simulink subsystem "Thermofluids_GS"  (R2025a)
settings: Solver=VariableStepAuto  StartTime=0.0  StopTime=10.0  RelTol=1e-3
settings Model: Creator=Adam  LastModifiedBy=MW

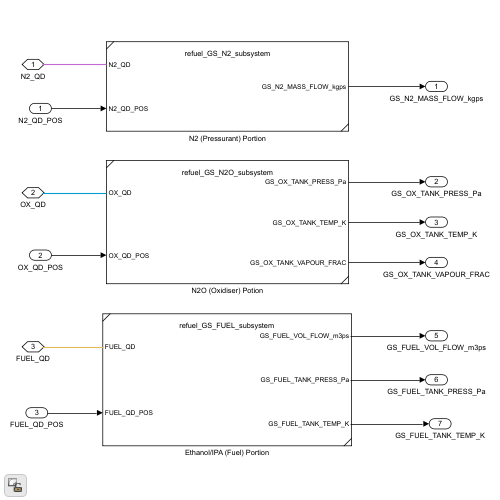
[thumbnail: Simulink's stored preview of the top-level diagram]
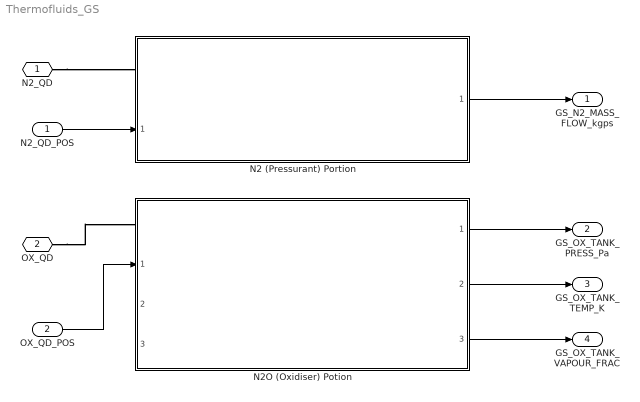
== system Thermofluids_GS ==
  N2_QD_POS : Inport
  OX_QD_POS : Inport  Port=2
  N2 (Pressurant) Portion : Subsystem  ReferencedSubsystem=refuel_GS_N2_subsystem
      settings: PortSchema="{\"entries\":[{\"content\":{\"sides\":[{\"content\":{\"connectorIds\":[\"LConn1\",\"In1\"]},\"type\":\"ConnectorPlacement.EquallySpacedRectSide\",\"uuid\":\"80a1b4a4-a86f-460b-b4b9-f1e834cc0a6f\"},{\"content\":{\"connectorIds\":[\"Out1\"],\"side\":\"RIGHT\"},\"type\":\"ConnectorPlacement.EquallySpacedRectSide\",\"uuid\":\"7a691a14-4b0a-4077-9abf-8e4fa479ec3d\"},{\"content\":{\"side\":\"TOP\"},\"type\":\"ConnectorPlacement.EquallySpacedRectSide\",\"uuid\":\"b8dd7e20-acb6-44c1-83ed-0b89a390ff72\"}]},\"type\":\"ConnectorPlacement.EquallySpacedConnector\",\"uuid\":\"2e88b817-b41b-4786-aed1-deff05c2a84d\"}],\"packageUris\":[\"http://schema.mathworks.com/mf0/Connector/R2020b\"],\"version\":\"1.0\"}"
  N2O (Oxidiser) Potion : Subsystem  ReferencedSubsystem=refuel_GS_N2O_subsystem
      settings: PortSchema="{\"entries\":[{\"content\":{\"sides\":[{\"content\":{\"connectorIds\":[\"LConn1\",\"In1\",\"In2\",\"In3\"]},\"type\":\"ConnectorPlacement.EquallySpacedRectSide\",\"uuid\":\"80a1b4a4-a86f-460b-b4b9-f1e834cc0a6f\"},{\"content\":{\"connectorIds\":[\"Out1\",\"Out2\",\"Out3\"],\"side\":\"RIGHT\"},\"type\":\"ConnectorPlacement.EquallySpacedRectSide\",\"uuid\":\"7a691a14-4b0a-4077-9abf-8e4fa479ec3d\"},{\"content\":{\"side\":\"TOP\"},\"type\":\"ConnectorPlacement.EquallySpacedRectSide\",\"uuid\":\"b8dd7e20-acb6-44c1-83ed-0b89a390ff72\"}]},\"type\":\"ConnectorPlacement.EquallySpacedConnector\",\"uuid\":\"2e88b817-b41b-4786-aed1-deff05c2a84d\"}],\"packageUris\":[\"http://schema.mathworks.com/mf0/Connector/R2020b\"],\"version\":\"1.0\"}"
  N2_QD : PMIOPort  Side=Left
  OX_QD : PMIOPort  Port=2  Side=Left
  GS_N2_MASS_FLOW_kgps : Outport
  GS_OX_TANK_PRESS_Pa : Outport  Port=2
  GS_OX_TANK_TEMP_K : Outport  Port=3
  GS_OX_TANK_VAPOUR_FRAC : Outport  Port=4
  wires:
  OX_QD_POS/1 -> N2O (Oxidiser) Potion/1
  N2O (Oxidiser) Potion/3 -> GS_OX_TANK_VAPOUR_FRAC/1
  N2 (Pressurant) Portion/1 -> GS_N2_MASS_FLOW_kgps/1
  N2_QD_POS/1 -> N2 (Pressurant) Portion/1
  N2O (Oxidiser) Potion/1 -> GS_OX_TANK_PRESS_Pa/1
  N2O (Oxidiser) Potion/2 -> GS_OX_TANK_TEMP_K/1
  connections:
  N2_QD/RConn1 -- N2 (Pressurant) Portion/LConn1
  OX_QD/RConn1 -- N2O (Oxidiser) Potion/LConn1
